simulink model "prach_shortFormat_fftShift"  (R2023b)
settings: Solver=FixedStepDiscrete  StartTime=0.0  StopTime=prach_short.SimulationTime  FixedStep=1  RelTol=1e-3  EnableMultiTasking=on
PreLoadFcn:
  | warning off Simulink:Commands:SetParamLinkChangeWarn
  | warning off Simulink:Commands:LoadMdlParameterizedLink
  | warning off Simulink:SL_SetParamLinkChangeWarn
  | warning off Simulink:SL_LoadMdlParameterizedLink
  | setup_prach_shortFormat;
InitFcn:
  | setup_prach_shortFormat;
StopFcn:
  | prach_post_run_script
values from neighbouring files (symbols this model uses):
  ConfigTable = [16 1 9,20,20,20,20,20,20,20,20,20 0 2 6 2 4 ... (first row only)    [ConfigIndexTable.m]
  NTxAnts = 4    [setup_prach_shortFormat.m]    (also in setup_prach_shortFormat_fftShift.m)
undefined symbols (not defined in the file or in its folder): AdvDSPBChannelOutDisplay, AdvDSPBDMemDisplay, BW, ControlDecode, display, dpoly, dspba, dspba_ChannelInVis, dspba_ChannelOutVis, dspba_internal_get_channel_ports, evalAionMaskParam, latency, PRACH_CC, PRACH_regs, prach_short, PrachLib, PrachLib_FFTshift, primtype, RemoveCP, Stream2BlockConv, UseDontCare, value, waveconfig
libraries: DSPBAPrim x397, DSPBAControl x16, DSPBAModelBus x7, DSPBABase x5, DSPBAUtilities x5, simulink x2, DSPBAVectorUtil x1, DspbAdvFftLibrary x1
(part 2 of 5)

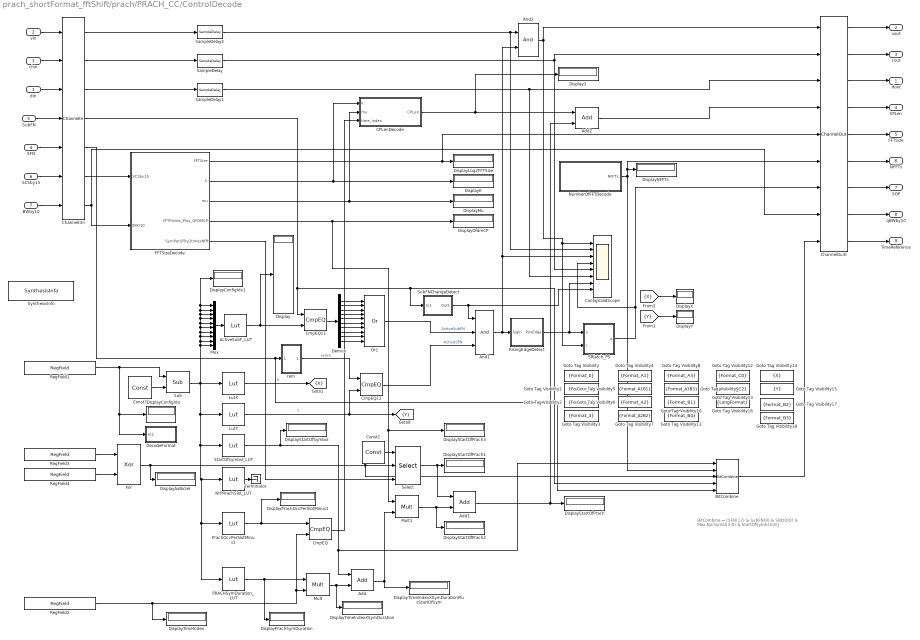
== system prach_shortFormat_fftShift/prach/PRACH_CC/ControlDecode ==
  note: BitCombine = [SFN(12) & SubFN(8) & SlotID(0) & Max.No.Symbl(3:0) & StartOfSymb(3:0)]
  din : Inport
  vin : Inport  Port=2
  chin : Inport  Port=3
  SFN : Inport  Port=4
  SubFN : Inport  Port=5
  SCSby15 : Inport  Port=6
  BWby10 : Inport  Port=7
  ActiveSubF_LUT : DSPBAPrim/Lut  primtype=lut  nInputs=1  nOutputs=1  omode=Inherit via internal rule  otype=sfix(16)  scale=2^-15  rndmethod=Unbiased  factor=1  satmethod=Symmetric  shift_vec=[0 1 2 -1]  value=ConfigTable(:,3:12)  inPortNames=[' '; ' ';]  outPortNames=[' ']  dspbaimage=dspba_prim.svg  text=fprintf('LUT');  style=Optimised  visibilities=8 + 1024  floatPrecision=float32_m23  version=20211007
  Add : DSPBAPrim/Add  primtype=add  nInputs=evalAionMaskParam(gcb,'value',1)  nOutputs=1  omode=Inherit via internal rule with word growth  otype=sfix(16)  scale=2^-15  rndmethod=Unbiased  factor=1  satmethod=Symmetric  shift_vec=[0 1 2 -1]  value=2  inPortNames=[' '; ' ';]  outPortNames=[' ']  dspbaimage=dspba_prim.svg  text=fprintf('+');  style=Optimised  visibilities=1032+2^17+2^18+2^19  genFPC=off  floatRounding=correct  advOptions=[]  version=20211007
  Add1 : DSPBAPrim/Add  primtype=add  nInputs=evalAionMaskParam(gcb,'value',1)  nOutputs=1  omode=Inherit via internal rule with word growth  otype=sfix(16)  scale=2^-15  rndmethod=Unbiased  factor=1  satmethod=Symmetric  shift_vec=[0 1 2 -1]  value=2  inPortNames=[' '; ' ';]  outPortNames=[' ']  dspbaimage=dspba_prim.svg  text=fprintf('+');  style=Optimised  visibilities=1032+2^17+2^18+2^19  genFPC=off  floatRounding=correct  advOptions=[]  version=20211007
  Add2 : DSPBAPrim/Add  primtype=add  nInputs=evalAionMaskParam(gcb,'value',1)  nOutputs=1  omode=Inherit via internal rule with word growth  otype=sfix(16)  scale=2^-15  rndmethod=Unbiased  factor=1  satmethod=Symmetric  shift_vec=[0 1 2 -1]  value=2  inPortNames=[' '; ' ';]  outPortNames=[' ']  dspbaimage=dspba_prim.svg  text=fprintf('+');  style=Optimised  visibilities=1032+2^17+2^18+2^19  genFPC=off  floatRounding=correct  advOptions=[]  version=20211007
  And1 : DSPBAPrim/And  primtype=and  nInputs=3  nOutputs=1  omode=Inherit via internal rule  otype=sfix(16)  scale=2^-15  rndmethod=Unbiased  factor=1  satmethod=Symmetric  shift_vec=[0 1 2 -1]  value=0  inPortNames=[' '; ' '; ' '; ' '; ' '; ' '; ' '; ' '; ' '; ' '; ' '; ' '; ' '; ' '; ' '; ' '; ]  outPortNames=[' ']  dspbaimage=dspba_prim.svg  text=fprintf('&');  style=Optimised  visibilities=8+2  version=20211007
  And2 : DSPBAPrim/And  primtype=and  nInputs=2  nOutputs=1  omode=Inherit via internal rule  otype=sfix(16)  scale=2^-15  rndmethod=Unbiased  factor=1  satmethod=Symmetric  shift_vec=[0 1 2 -1]  value=0  inPortNames=[' '; ' '; ' '; ' '; ' '; ' '; ' '; ' '; ' '; ' '; ' '; ' '; ' '; ' '; ' '; ' '; ]  outPortNames=[' ']  dspbaimage=dspba_prim.svg  text=fprintf('&');  style=Optimised  visibilities=8+2  version=20211007
  BitCombine : DSPBAPrim/BitCombine  primtype=bitcombine  nInputs=5  nOutputs=1  omode=Inherit via internal rule  otype=sfix(16)  scale=2^-15  rndmethod=Unbiased  factor=1  satmethod=Symmetric  shift_vec=[0 1 2 -1]  value=0  inPortNames=['l'; 'h';]  outPortNames=[' ']  dspbaimage=dspba_prim.svg  text=fprintf('[h,l]');  style=Optimised  visibilities=8+2  version=20211007
  CPLenDecode : Subsystem
      mask Display:
      | color('w');
      | image('dspba_prim.jpg');
      | port_label('output',1,'CPLen*nAnt');
      | port_label('input',1,'k');
      | port_label('input',2,'mu');
      | port_label('input',3,'time_index');
  ChannelI3n : DSPBAPrim/ChannelIn  primtype=channelin  nInputs=dspba_internal_get_channel_ports(gcb)  nOutputs=dspba_internal_get_channel_ports(gcb)  omode=Inherit via internal rule  otype=sfix(16)  scale=2^-15  rndmethod=Unbiased  factor=1  satmethod=Symmetric  shift_vec=[0 1 2 -1]  value=5  inPortNames=['v'; 'c'; '0'; '1'; '2'; '3'; '4'; '5'; '6'; '7'; '8'; '9'; 'A'; 'B'; 'D'; 'E'; 'F'; 'G'; 'H'; 'I'; 'J'; 'K'; 'L'; 'M'; 'N'; 'O'; 'P'; 'Q'; 'R'; 'S'; 'T'; 'U'; 'W'; 'X'; 'Y'; 'Z']  outPortNames=['v'; 'c'; '0'; '1'; '2'; '3'; '4'; '5'; '6'; '7'; '8'; '9'; 'A'; 'B'; 'D'; 'E'; 'F'; 'G'; 'H'; 'I'; 'J'; 'K'; 'L'; 'M'; 'N'; 'O'; 'P'; 'Q'; 'R'; 'S'; 'T'; 'U'; 'W'; 'X'; 'Y'; 'Z']  dspbaimage=dspba_prim_channel_tall.svg  text=fprintf('In');  style=Optimised  dataSignals=5  foldingEnabled=off  channels=1  sampleRate=200  packetBeginPresent=off  packetBeginEnabled=off  visibilities=dspba_ChannelInVis(gcb)  scheduleOrigin=on  version=20211214
  ChannelOu3t : DSPBAPrim/ChannelOut  primtype=channelout  nInputs=dspba_internal_get_channel_ports(gcb)  nOutputs=dspba_internal_get_channel_ports(gcb)  omode=Inherit via internal rule  otype=sfix(16)  scale=2^-15  rndmethod=Unbiased  factor=1  satmethod=Symmetric  shift_vec=[0 1 2 -1]  value=7  inPortNames=['v'; 'c'; '0'; '1'; '2'; '3'; '4'; '5'; '6'; '7'; '8'; '9'; 'A'; 'B'; 'D'; 'E'; 'F'; 'G'; 'H'; 'I'; 'J'; 'K'; 'L'; 'M'; 'N'; 'O'; 'P'; 'Q'; 'R'; 'S'; 'T'; 'U'; 'W'; 'X'; 'Y'; 'Z']  outPortNames=['v'; 'c'; '0'; '1'; '2'; '3'; '4'; '5'; '6'; '7'; '8'; '9'; 'A'; 'B'; 'D'; 'E'; 'F'; 'G'; 'H'; 'I'; 'J'; 'K'; 'L'; 'M'; 'N'; 'O'; 'P'; 'Q'; 'R'; 'S'; 'T'; 'U'; 'W'; 'X'; 'Y'; 'Z']  dspbaimage=dspba_prim_channel_tall.svg  text=fprintf('Out%s', AdvDSPBChannelOutDisplay(latency));  style=Optimised  dataSignals=7  foldingEnabled=off  channels=1  sampleRate=200  packetBeginPresent=off  packetBeginEnabled=off  visibilities=dspba_ChannelOutVis(gcb)  latency=17  version=20211214
  CmpEQ : DSPBAPrim/CmpEQ  primtype=cmpeq  nInputs=2  nOutputs=1  omode=boolean  otype=sfix(16)  scale=2^-15  rndmethod=Unbiased  factor=1  satmethod=Symmetric  shift_vec=[0 1 2 -1]  value=0  inPortNames=[' '; ' ';]  outPortNames=[' ']  dspbaimage=dspba_prim.svg  text=fprintf('==');  style=Optimised  visibilities=0  advOptions=[]  version=20211007
  CmpEQ11 : DSPBAPrim/CmpEQ  primtype=cmpeq  nInputs=2  nOutputs=1  omode=boolean  otype=sfix(16)  scale=2^-15  rndmethod=Unbiased  factor=1  satmethod=Symmetric  shift_vec=[0 1 2 -1]  value=0  inPortNames=[' '; ' ';]  outPortNames=[' ']  dspbaimage=dspba_prim.svg  text=fprintf('==');  style=Optimised  visibilities=0  advOptions=[]  version=20211007
  CmpEQ12 : DSPBAPrim/CmpEQ  primtype=cmpeq  nInputs=2  nOutputs=1  omode=boolean  otype=sfix(16)  scale=2^-15  rndmethod=Unbiased  factor=1  satmethod=Symmetric  shift_vec=[0 1 2 -1]  value=0  inPortNames=[' '; ' ';]  outPortNames=[' ']  dspbaimage=dspba_prim.svg  text=fprintf('==');  style=Optimised  visibilities=0  advOptions=[]  version=20211007
  ConfigValidScope : Scope  NumInputPorts=8
  Const1 : DSPBAPrim/Const  primtype=const  nInputs=0  nOutputs=1  omode=Inherit via internal rule  otype=sfix(16)  scale=2^-15  rndmethod=Unbiased  factor=1  satmethod=Symmetric  shift_vec=[0 1 2 -1]  value=0  inPortNames=['+'; '+';]  outPortNames=[' ']  dspbaimage=dspba_prim.svg  text=fprintf('%s', num2str(value));  style=Optimised  visibilities=8 + 1024  floatPrecision=float32_m23  warnSaturation=on  version=20211007  SampleTime=inf
  Const3 : DSPBAPrim/Const  primtype=const  nInputs=0  nOutputs=1  omode=Inherit via internal rule  otype=sfix(16)  scale=2^-15  rndmethod=Unbiased  factor=1  satmethod=Symmetric  shift_vec=[0 1 2 -1]  value=67  inPortNames=['+'; '+';]  outPortNames=[' ']  dspbaimage=dspba_prim.svg  text=fprintf('%s', num2str(value));  style=Optimised  visibilities=8 + 1024  floatPrecision=float32_m23  warnSaturation=on  version=20211007  SampleTime=inf
  DecodeFormat : Subsystem
  Demux : Demux  Outputs=10
  Display : Display
  Display3 : Display
  DisplayAxBxSel : Display
  DisplayConfigIdx : Display
  DisplayConfigIdx1 : Display
  DisplayK : Display
  DisplayLog2FFTSize : Display
  DisplayMu : Display
  DisplayNFFTs : Display
  DisplayOfdmCP : Display
  DisplayPrachOccPerSlotMinus1 : Display
  DisplayPrachSymDuration : Display
  DisplayStartOfPrach{,1..3} (4 alike) : Display
  DisplayStartOfSymbol : Display
  DisplayTimeIndex : Display
  DisplayTimeIndexXSymDuration : Display
  DisplayTimeIndexXSymDurationPlusStartOfSym : Display
  DisplayX : Display
  DisplayY : Display
  FFTSizeDecode : Subsystem
      mask Display:
      | color('w');
      | image('dspba_prim.jpg');
      | port_label('output',1,'log2(FFT size)');
      | port_label('output',2,'k');
      | port_label('output',3,'mu');
      | port_label('output',4,'FFTPoints+OFDM_CP');
      | port_label('output',5,'SymPerSF/2*Nfft');
      | port_label('input',1,'SCS/15');
      | port_label('input',2,'BW/10');
  Goto Tag Visibility : GotoTagVisibility  GotoTag=Format_0
  Goto Tag Visibility1 : GotoTagVisibility  GotoTag=Format_1
  Goto Tag Visibility10 : GotoTagVisibility  GotoTag=Format_B1
  Goto Tag Visibility11 : GotoTagVisibility  GotoTag=Format_B4
  Goto Tag Visibility12 : GotoTagVisibility  GotoTag=Format_C0
  Goto Tag Visibility13 : GotoTagVisibility  GotoTag=Format_C2
  Goto Tag Visibility14 : GotoTagVisibility  GotoTag=X
  Goto Tag Visibility15 : GotoTagVisibility  GotoTag=Y
  Goto Tag Visibility16 : GotoTagVisibility  GotoTag=LongFormat
  Goto Tag Visibility17 : GotoTagVisibility  GotoTag=Format_B2
  Goto Tag Visibility18 : GotoTagVisibility  GotoTag=Format_B3
  Goto Tag Visibility2 : GotoTagVisibility  GotoTag=Format_2
  Goto Tag Visibility3 : GotoTagVisibility  GotoTag=Format_3
  Goto Tag Visibility4 : GotoTagVisibility  GotoTag=Format_A1
  Goto Tag Visibility5 : GotoTagVisibility  GotoTag=Format_A1B1
  Goto Tag Visibility6 : GotoTagVisibility  GotoTag=Format_A2
  Goto Tag Visibility7 : GotoTagVisibility  GotoTag=Format_A2B2
  Goto Tag Visibility8 : GotoTagVisibility  GotoTag=Format_A3
  Goto Tag Visibility9 : GotoTagVisibility  GotoTag=Format_A3B3
  LutX : DSPBAPrim/Lut  primtype=lut  nInputs=1  nOutputs=1  omode=Inherit via internal rule  otype=sfix(16)  scale=2^-15  rndmethod=Unbiased  factor=1  satmethod=Symmetric  shift_vec=[0 1 2 -1]  value=ConfigTable(:,1)  inPortNames=[' '; ' ';]  outPortNames=[' ']  dspbaimage=dspba_prim.svg  text=fprintf('LUT');  style=Optimised  visibilities=8 + 1024  floatPrecision=float32_m23  version=20211007
  LutY : DSPBAPrim/Lut  primtype=lut  nInputs=1  nOutputs=1  omode=Inherit via internal rule  otype=sfix(16)  scale=2^-15  rndmethod=Unbiased  factor=1  satmethod=Symmetric  shift_vec=[0 1 2 -1]  value=ConfigTable(:,2)  inPortNames=[' '; ' ';]  outPortNames=[' ']  dspbaimage=dspba_prim.svg  text=fprintf('LUT');  style=Optimised  visibilities=8 + 1024  floatPrecision=float32_m23  version=20211007
  Mult : DSPBAPrim/Mult  primtype=mult  nInputs=2  nOutputs=1  omode=Inherit via internal rule  otype=sfix(16)  scale=2^-15  rndmethod=Unbiased  factor=1  satmethod=Symmetric  shift_vec=[0 1 2 -1]  value=0  inPortNames=[' '; ' ';]  outPortNames=[' ']  dspbaimage=dspba_prim.svg  text=fprintf('X');  style=Optimised  visibilities=8+2^18+2^19  floatPrecision=float32_m23  floatRounding=correct  advOptions=[]  version=20211007
  Mult1 : DSPBAPrim/Mult  primtype=mult  nInputs=2  nOutputs=1  omode=Inherit via internal rule  otype=sfix(16)  scale=2^-15  rndmethod=Unbiased  factor=1  satmethod=Symmetric  shift_vec=[0 1 2 -1]  value=0  inPortNames=[' '; ' ';]  outPortNames=[' ']  dspbaimage=dspba_prim.svg  text=fprintf('X');  style=Optimised  visibilities=8+2^18+2^19  floatPrecision=float32_m23  floatRounding=correct  advOptions=[]  version=20211007
  Mux : Mux  Inputs=10
  NrPRrachSlot_LUT : DSPBAPrim/Lut  primtype=lut  nInputs=1  nOutputs=1  omode=Inherit via internal rule  otype=sfix(16)  scale=2^-15  rndmethod=Unbiased  factor=1  satmethod=Symmetric  shift_vec=[0 1 2 -1]  value=ConfigTable(:,14)  inPortNames=[' '; ' ';]  outPortNames=[' ']  dspbaimage=dspba_prim.svg  text=fprintf('LUT');  style=Optimised  visibilities=8 + 1024  floatPrecision=float32_m23  version=20211007
  NumberOfFFTDecode : Subsystem
      mask Display:
      | color('w');
      | image('dspba_prim.jpg');
      | port_label('output',1,'Number of FFTs');
  Or1 : DSPBAPrim/Or  primtype=or  nInputs=10  nOutputs=1  omode=Inherit via internal rule  otype=sfix(16)  scale=2^-15  rndmethod=Unbiased  factor=1  satmethod=Symmetric  shift_vec=[0 1 2 -1]  value=0  inPortNames=[' '; ' '; ' '; ' '; ' '; ' '; ' '; ' '; ' '; ' '; ' '; ' '; ' '; ' '; ' '; ' '; ]  outPortNames=[' ']  dspbaimage=dspba_prim.svg  text=fprintf('|');  style=Optimised  visibilities=8+2  version=20211007
  PRACHSymDuration_LUT : DSPBAPrim/Lut  primtype=lut  nInputs=1  nOutputs=1  omode=Inherit via internal rule  otype=sfix(16)  scale=2^-15  rndmethod=Unbiased  factor=1  satmethod=Symmetric  shift_vec=[0 1 2 -1]  value=ConfigTable(:,16)  inPortNames=[' '; ' ';]  outPortNames=[' ']  dspbaimage=dspba_prim.svg  text=fprintf('LUT');  style=Optimised  visibilities=8 + 1024  floatPrecision=float32_m23  version=20211007
  PrachOccPerSlotMinus1 : DSPBAPrim/Lut  primtype=lut  nInputs=1  nOutputs=1  omode=Inherit via internal rule  otype=sfix(16)  scale=2^-15  rndmethod=Unbiased  factor=1  satmethod=Symmetric  shift_vec=[0 1 2 -1]  value=ConfigTable(:,15)-1  inPortNames=[' '; ' ';]  outPortNames=[' ']  dspbaimage=dspba_prim.svg  text=fprintf('LUT');  style=Optimised  visibilities=8 + 1024  floatPrecision=float32_m23  version=20211007
  RegField1 : DSPBAModelBus/RegField  reg_name=PRACH_regs(InstanceNumber).PRACH_config_index_addr  reg_rwmode=Read/Write  reg_msb=7  reg_lsb=0  reg_mode=Specify via dialog  reg_type=uint(8)  reg_scale=2^0  reg_init=PRACH_regs(InstanceNumber).PRACH_config_index  reg_desc=PRACH_regs(InstanceNumber).PRACH_config_index_string  reg_modal=off  reg_desc0=0  reg_desc1=0  reg_desc2=0  reg_desc3=0  reg_desc4=0  reg_desc5=0  reg_desc6=0  reg_desc7=0  reg_addr=8  SampleTime=-1  version=20090407
  RegField2 : DSPBAModelBus/RegField  reg_name=PRACH_regs(InstanceNumber).PRACH_time_index_addr  reg_rwmode=Read/Write  reg_msb=2  reg_lsb=0  reg_mode=Specify via dialog  reg_type=uint(3)  reg_scale=2^0  reg_init=PRACH_regs(InstanceNumber).PRACH_time_index  reg_desc=PRACH_regs(InstanceNumber).PRACH_time_index_string  reg_modal=off  reg_desc0=0  reg_desc1=0  reg_desc2=0  reg_desc3=0  reg_desc4=0  reg_desc5=0  reg_desc6=0  reg_desc7=0  reg_addr=9  SampleTime=-1  version=20090407
  RegField3 : DSPBAModelBus/RegField  reg_name=PRACH_regs(InstanceNumber).PRACH_NRPRACHSlot_addr  reg_rwmode=Read/Write  reg_msb=0  reg_lsb=0  reg_mode=Specify via dialog  reg_type=uint(1)  reg_scale=2^0  reg_init=PRACH_regs(InstanceNumber).PRACH_NRPRACHSlot  reg_desc=PRACH_regs(InstanceNumber).PRACH_NRPRACHSlot_string  reg_modal=off  reg_desc0=0  reg_desc1=0  reg_desc2=0  reg_desc3=0  reg_desc4=0  reg_desc5=0  reg_desc6=0  reg_desc7=0  reg_addr=10  SampleTime=-1  version=20090407
  RegField4 : DSPBAModelBus/RegField  reg_name=PRACH_regs(InstanceNumber).PRACH_ActivePRACHSlot_addr  reg_rwmode=Read/Write  reg_msb=0  reg_lsb=0  reg_mode=Specify via dialog  reg_type=uint(1)  reg_scale=2^0  reg_init=PRACH_regs(InstanceNumber).PRACH_ActivePRACHSlot  reg_desc=PRACH_regs(InstanceNumber).PRACH_ActivePRACHSlot_string  reg_modal=off  reg_desc0=0  reg_desc1=0  reg_desc2=0  reg_desc3=0  reg_desc4=0  reg_desc5=0  reg_desc6=0  reg_desc7=0  reg_addr=11  SampleTime=-1  version=20090407
  RisingEdgeDetect : Subsystem
  SRlatch_PS : Subsystem  AncestorBlock=DSPBAControl/SRlatch_PS  mask(SetResetLatchPrioritySet){}
      mask help: DSP Builder offers two single-cycle latency latch subsystems for common operations for the valid signal, latching with set and reset. The SRlatch block gives priority to the reset input signal; the SRlatch_PS block gives priority to the set input signal. In both blocks, if set and reset inputs are both zero the current output state is maintained.
      mask Help: helpview(dspba.GetHelp('SRlatch_PS'));
      mask Display:
      | color('w');
      | image('dspba_prim_masked.png');
      | fprintf('SRlatch\nPriority\nSet');
      | port_label('input',1,'s');
      | port_label('input',2,'r');
      | port_label('output',1,'q');
  SampleDelay : DSPBAPrim/SampleDelay  primtype=sampdelay  nInputs=1  nOutputs=1  omode=Inherit via internal rule  otype=sfix(16)  scale=2^-15  rndmethod=Unbiased  factor=1  satmethod=Symmetric  shift_vec=[0 1 2 -1]  floatPrecision=float32_m23  value=1  inPortNames=[' '; ' ';]  outPortNames=[' ']  dspbaimage=dspba_prim.svg  text=dpoly(1, eye(1,value+1), 'z')  style=Optimised  visibilities=8 + 1024 + 2^17 + 2^18  flexible=off  slackgroup=0  augmented=0  version=20211007  advOptions=[]
  SampleDelay1 : DSPBAPrim/SampleDelay  primtype=sampdelay  nInputs=1  nOutputs=1  omode=Inherit via internal rule  otype=sfix(16)  scale=2^-15  rndmethod=Unbiased  factor=1  satmethod=Symmetric  shift_vec=[0 1 2 -1]  floatPrecision=float32_m23  value=1  inPortNames=[' '; ' ';]  outPortNames=[' ']  dspbaimage=dspba_prim.svg  text=dpoly(1, eye(1,value+1), 'z')  style=Optimised  visibilities=8 + 1024 + 2^17 + 2^18  flexible=off  slackgroup=0  augmented=0  version=20211007  advOptions=[]
  SampleDelay2 : DSPBAPrim/SampleDelay  primtype=sampdelay  nInputs=1  nOutputs=1  omode=Inherit via internal rule  otype=sfix(16)  scale=2^-15  rndmethod=Unbiased  factor=1  satmethod=Symmetric  shift_vec=[0 1 2 -1]  floatPrecision=float32_m23  value=1  inPortNames=[' '; ' ';]  outPortNames=[' ']  dspbaimage=dspba_prim.svg  text=dpoly(1, eye(1,value+1), 'z')  style=Optimised  visibilities=8 + 1024 + 2^17 + 2^18  flexible=off  slackgroup=0  augmented=0  version=20211007  advOptions=[]
  Select : DSPBAPrim/Select  primtype=select  nInputs=str2num(get_param(gcb,'value'))*2+1  nOutputs=1  omode=Inherit via internal rule  otype=sfix(16)  scale=2^-15  rndmethod=Unbiased  factor=1  satmethod=Symmetric  shift_vec=[0 1 2 -1]  value=1  inPortNames=['d'; '0'; 'a'; '1'; 'b'; '2'; 'c'; '3'; 'd'; '4'; 'e'; '5'; 'f'; '6'; 'g'; '7'; 'h'; '8'; 'i'; '9'; 'j']  outPortNames=[' ']  dspbaimage=dspba_prim_tall.svg  text=fprintf('%s', primtype);  style=Optimised  visibilities=8 + 1024  version=20211007
  StartOfSymbol_LUT : DSPBAPrim/Lut  primtype=lut  nInputs=1  nOutputs=1  omode=Inherit via internal rule  otype=sfix(16)  scale=2^-15  rndmethod=Unbiased  factor=1  satmethod=Symmetric  shift_vec=[0 1 2 -1]  value=ConfigTable(:,13)  inPortNames=[' '; ' ';]  outPortNames=[' ']  dspbaimage=dspba_prim.svg  text=fprintf('LUT');  style=Optimised  visibilities=8 + 1024  floatPrecision=float32_m23  version=20211007
  Sub : DSPBAPrim/Sub  primtype=sub  nInputs=2  nOutputs=1  omode=Specify via dialog  otype=uint(8)  scale=1  rndmethod=Unbiased  factor=1  satmethod=Symmetric  shift_vec=[0 1 2 -1]  value=0  inPortNames=['+'; '-';]  outPortNames=[' ']  dspbaimage=dspba_prim.svg  text=fprintf('-');  style=Optimised  visibilities=8+2^17+2^18  floatRounding=correct  advOptions=[]  version=20211007
  SubFNChangeDetect : Subsystem
  SynthesisInfo : DSPBAPrim/SynthesisInfo  primtype=synthinfo  nInputs=0  nOutputs=0  omode=Inherit via internal rule  otype=sfix(16)  scale=2^-15  rndmethod=Truncate  factor=1  satmethod=Symmetric  shift_vec=[0 1 2 -1]  value=99  inPortNames=[' '; ' ';]  outPortNames=[' ']  dspbaimage=dspba_prim_ctrl.jpg  text=fprintf('Style=%s', style);  style=Scheduled  visibilities=2^17+2^18+2^19+2^20+2^21+2^22+2^23+2^24  constraintPair=None  constraintRelation=>  constraintLimit=2  modelRefSign=+  modelRef=''  showSchedule=off  simulationMode=Use Global Value  resetMinimization=Conditional - On for ChannelIn/Out only  version=20220106
  Terminator : Terminator
  Xor : DSPBAPrim/Xor  primtype=xor  nInputs=2  nOutputs=1  omode=Inherit via internal rule  otype=sfix(16)  scale=2^-15  rndmethod=Unbiased  factor=1  satmethod=Symmetric  shift_vec=[0 1 2 -1]  value=0  inPortNames=[' '; ' '; ' '; ' '; ' '; ' '; ' '; ' '; ' '; ' '; ' '; ' '; ' '; ' '; ' '; ' '; ]  outPortNames=[' ']  dspbaimage=dspba_prim.svg  text=fprintf('^');  style=Optimised  visibilities=8+2  version=20211007
  rem : Subsystem
  dout : Outport  VectorParamsAs1DForOutWhenUnconnected=off
  vout : Outport  Port=2  VectorParamsAs1DForOutWhenUnconnected=off
  cout : Outport  Port=3  VectorParamsAs1DForOutWhenUnconnected=off
  CPLen : Outport  Port=4  VectorParamsAs1DForOutWhenUnconnected=off
  FFTSize : Outport  Port=5  VectorParamsAs1DForOutWhenUnconnected=off
  NFFTs : Outport  Port=6  VectorParamsAs1DForOutWhenUnconnected=off
  SOP : Outport  Port=7  VectorParamsAs1DForOutWhenUnconnected=off
  qBWby10 : Outport  Port=8  VectorParamsAs1DForOutWhenUnconnected=off
  TimeReference : Outport  Port=9  VectorParamsAs1DForOutWhenUnconnected=off
  tag scope: X=scoped, Y=scoped
  wires:
  LutY/1 -> [Y], CmpEQ12/2  "Y"
  LutX/1 -> [X]  "X"
  Mux/1 -> ActiveSubF_LUT/1
  ActiveSubF_LUT/1 -> CmpEQ11/2, Display/1
  ChannelI3n/3 -> SampleDelay1/1
  ChannelI3n/4 -> SubFNChangeDetect/1(In1), BitCombine/4, CmpEQ11/1
  din/1 -> ChannelI3n/3
  chin/1 -> ChannelI3n/2
  vin/1 -> ChannelI3n/1
  ChannelI3n/2 -> SampleDelay/1
  ChannelOu3t/3 -> dout/1
  ChannelOu3t/2 -> cout/1
  ChannelOu3t/1 -> vout/1
  SampleDelay2/1 -> ConfigValidScope/2, And2/1
  RegField1/1 -> DisplayConfigIdx/1, DecodeFormat/1(In1), Sub/1
  ChannelI3n/5 -> BitCombine/5, rem/1(SFN)
  rem/1(rem) -> CmpEQ12/1  "remX"
  CmpEQ12/1 -> And1/3  "ActiveSFN"
  And2/1 -> SRlatch_PS/2(r), ConfigValidScope/1, ChannelOu3t/1
  Demux/1 -> Or1/1
  Demux/2 -> Or1/2
  Demux/3 -> Or1/3
  Demux/4 -> Or1/4
  Demux/5 -> Or1/5
  Demux/6 -> Or1/6
  Demux/7 -> Or1/7
  Demux/8 -> Or1/8
  Demux/9 -> Or1/9
  Demux/10 -> Or1/10
  CmpEQ11/1 -> Demux/1
  Sub/1 -> LutX/1, PRACHSymDuration_LUT/1, PrachOccPerSlotMinus1/1, NrPRrachSlot_LUT/1, StartOfSymbol_LUT/1, LutY/1, DisplayConfigIdx1/1, Mux/1, Mux/2, Mux/3, Mux/4, Mux/5, Mux/6, Mux/7, Mux/8, Mux/9, Mux/10
  Const3/1 -> Sub/2
  SubFN/1 -> ChannelI3n/4
  SFN/1 -> ChannelI3n/5
  CPLenDecode/1(CPLen) -> Add2/1, Display3/1
  ChannelOu3t/4 -> CPLen/1
  ChannelOu3t/5 -> FFTSize/1
  SCSby15/1 -> ChannelI3n/6
  BWby10/1 -> ChannelI3n/7
  ChannelI3n/6 -> FFTSizeDecode/1(SCSby15)
  ChannelI3n/7 -> FFTSizeDecode/2(BW/10), ChannelOu3t/8
  FFTSizeDecode/2(k) -> CPLenDecode/1(k), DisplayK/1
  FFTSizeDecode/3(mu) -> CPLenDecode/2(mu), DisplayMu/1
  [X] -> DisplayX/1
  [Y] -> DisplayY/1
  NumberOfFFTDecode/1(NFFTs) -> ChannelOu3t/6, DisplayNFFTs/1, BitCombine/2
  ChannelOu3t/6 -> NFFTs/1
  And1/1 -> RisingEdgeDetect/1(SigIn), And2/2, ConfigValidScope/3
  Or1/1 -> And1/2  "ActiveSubFN"
  ChannelOu3t/7 -> SOP/1
  RisingEdgeDetect/1(PosEdge) -> ConfigValidScope/7, SRlatch_PS/1(s)
  FFTSizeDecode/1(FFTSize) -> DisplayLog2FFTSize/1, ChannelOu3t/5
  FFTSizeDecode/4(FFTPoints_Plus_OFDMCP) -> Mult1/1, DisplayStartOfPrach3/1, DisplayOfdmCP/1
  RegField2/1 -> DisplayTimeIndex/1, CmpEQ/2, Mult/2
  PRACHSymDuration_LUT/1 -> DisplayPrachSymDuration/1, Mult/1
  Mult/1 -> DisplayTimeIndexXSymDuration/1, Add/2
  StartOfSymbol_LUT/1 -> DisplayStartOfSymbol/1, BitCombine/1, Add/1
  Add/1 -> Mult1/2, DisplayTimeIndexXSymDurationPlusStartOfSym/1
  Mult1/1 -> DisplayStartOfPrach2/1, Add1/2
  FFTSizeDecode/5(SymPerSFby2timesNfft) -> Select/3
  RegField3/1 -> Xor/1
  RegField4/1 -> Xor/2
  Select/1 -> DisplayStartOfPrach1/1, Add1/1
  Xor/1 -> DisplayAxBxSel/1, BitCombine/3, Select/2
  Const1/1 -> Select/1
  Add1/1 -> Add2/2, DisplayStartOfPrach/1
  Add2/1 -> ChannelOu3t/4
  ChannelOu3t/8 -> qBWby10/1
  SRlatch_PS/1(q) -> ChannelOu3t/7, ConfigValidScope/4
  CmpEQ/1 -> CPLenDecode/3(time_index)
  NrPRrachSlot_LUT/1 -> Terminator/1
  PrachOccPerSlotMinus1/1 -> CmpEQ/1, DisplayPrachOccPerSlotMinus1/1
  BitCombine/1 -> ChannelOu3t/9
  ChannelOu3t/9 -> TimeReference/1
  SubFNChangeDetect/1(Out1) -> ConfigValidScope/8, And1/1
  SampleDelay/1 -> ChannelOu3t/2, ConfigValidScope/5
  SampleDelay1/1 -> ConfigValidScope/6, ChannelOu3t/3
  ChannelI3n/1 -> SampleDelay2/1

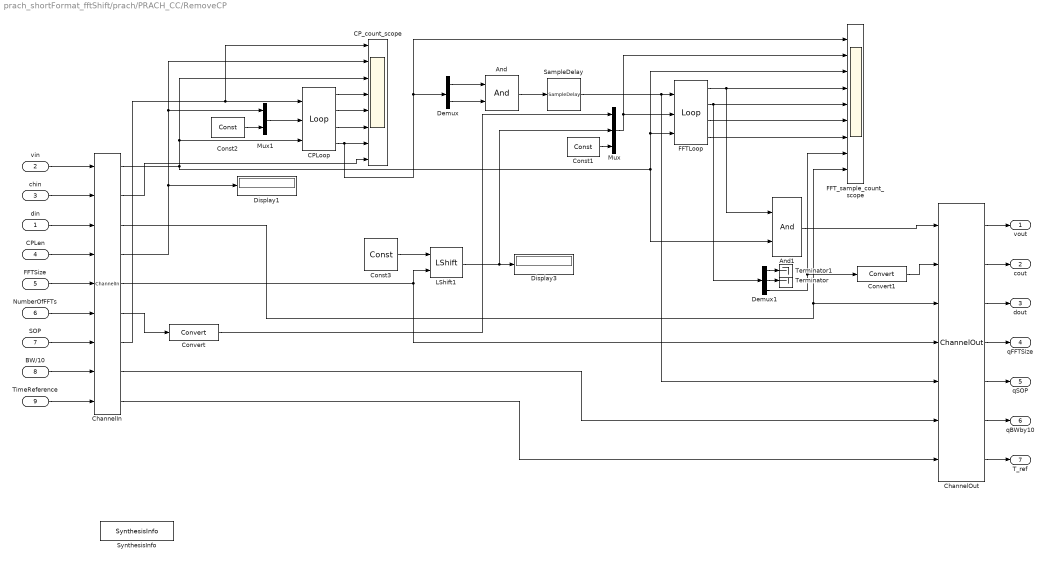
== system prach_shortFormat_fftShift/prach/PRACH_CC/RemoveCP ==
  din : Inport
  vin : Inport  Port=2
  chin : Inport  Port=3
  CPLen : Inport  Port=4
  FFTSize : Inport  Port=5
  NumberOfFFTs : Inport  Port=6
  SOP : Inport  Port=7
  BW/10 : Inport  Port=8
  TimeReference : Inport  Port=9
  And : DSPBAPrim/And  primtype=and  nInputs=2  nOutputs=1  omode=Inherit via internal rule  otype=sfix(16)  scale=2^-15  rndmethod=Unbiased  factor=1  satmethod=Symmetric  shift_vec=[0 1 2 -1]  value=0  inPortNames=[' '; ' '; ' '; ' '; ' '; ' '; ' '; ' '; ' '; ' '; ' '; ' '; ' '; ' '; ' '; ' '; ]  outPortNames=[' ']  dspbaimage=dspba_prim.svg  text=fprintf('&');  style=Optimised  visibilities=8+2  version=20211007
  And1 : DSPBAPrim/And  primtype=and  nInputs=2  nOutputs=1  omode=Inherit via internal rule  otype=sfix(16)  scale=2^-15  rndmethod=Unbiased  factor=1  satmethod=Symmetric  shift_vec=[0 1 2 -1]  value=0  inPortNames=[' '; ' '; ' '; ' '; ' '; ' '; ' '; ' '; ' '; ' '; ' '; ' '; ' '; ' '; ' '; ' '; ]  outPortNames=[' ']  dspbaimage=dspba_prim.svg  text=fprintf('&');  style=Optimised  visibilities=8+2  version=20211007
  CPLoop : DSPBAPrim/Loop  primtype=loop  nInputs=3  nOutputs=4  omode=Inherit via internal rule  otype=sfix(16)  scale=2^-15  rndmethod=Unbiased  factor=1  satmethod=Symmetric  shift_vec=[0 1 2 -1]  value=[zeros(16, 1)]  inPortNames=['g'; 'c'; 'e']  outPortNames=['v'; 'q'; 'f'; 'l']  dspbaimage=dspba_prim_tall.svg  text=fprintf('loop');  style=Optimised  visibilities=0  version=20211007
  CP_count_scope : Scope  NumInputPorts=8
  ChannelIn : DSPBAPrim/ChannelIn  primtype=channelin  nInputs=dspba_internal_get_channel_ports(gcb)  nOutputs=dspba_internal_get_channel_ports(gcb)  omode=Inherit via internal rule  otype=sfix(16)  scale=2^-15  rndmethod=Unbiased  factor=1  satmethod=Symmetric  shift_vec=[0 1 2 -1]  value=7  inPortNames=['v'; 'c'; '0'; '1'; '2'; '3'; '4'; '5'; '6'; '7'; '8'; '9'; 'A'; 'B'; 'D'; 'E'; 'F'; 'G'; 'H'; 'I'; 'J'; 'K'; 'L'; 'M'; 'N'; 'O'; 'P'; 'Q'; 'R'; 'S'; 'T'; 'U'; 'W'; 'X'; 'Y'; 'Z']  outPortNames=['v'; 'c'; '0'; '1'; '2'; '3'; '4'; '5'; '6'; '7'; '8'; '9'; 'A'; 'B'; 'D'; 'E'; 'F'; 'G'; 'H'; 'I'; 'J'; 'K'; 'L'; 'M'; 'N'; 'O'; 'P'; 'Q'; 'R'; 'S'; 'T'; 'U'; 'W'; 'X'; 'Y'; 'Z']  dspbaimage=dspba_prim_channel_tall.svg  text=fprintf('In');  style=Optimised  dataSignals=7  foldingEnabled=off  channels=1  sampleRate=200  packetBeginPresent=off  packetBeginEnabled=off  visibilities=dspba_ChannelInVis(gcb)  scheduleOrigin=on  version=20211214
  ChannelOut : DSPBAPrim/ChannelOut  primtype=channelout  nInputs=dspba_internal_get_channel_ports(gcb)  nOutputs=dspba_internal_get_channel_ports(gcb)  omode=Inherit via internal rule  otype=sfix(16)  scale=2^-15  rndmethod=Unbiased  factor=1  satmethod=Symmetric  shift_vec=[0 1 2 -1]  value=5  inPortNames=['v'; 'c'; '0'; '1'; '2'; '3'; '4'; '5'; '6'; '7'; '8'; '9'; 'A'; 'B'; 'D'; 'E'; 'F'; 'G'; 'H'; 'I'; 'J'; 'K'; 'L'; 'M'; 'N'; 'O'; 'P'; 'Q'; 'R'; 'S'; 'T'; 'U'; 'W'; 'X'; 'Y'; 'Z']  outPortNames=['v'; 'c'; '0'; '1'; '2'; '3'; '4'; '5'; '6'; '7'; '8'; '9'; 'A'; 'B'; 'D'; 'E'; 'F'; 'G'; 'H'; 'I'; 'J'; 'K'; 'L'; 'M'; 'N'; 'O'; 'P'; 'Q'; 'R'; 'S'; 'T'; 'U'; 'W'; 'X'; 'Y'; 'Z']  dspbaimage=dspba_prim_channel_tall.svg  text=fprintf('Out%s', AdvDSPBChannelOutDisplay(latency));  style=Optimised  dataSignals=5  foldingEnabled=off  channels=1  sampleRate=200  packetBeginPresent=off  packetBeginEnabled=off  visibilities=dspba_ChannelOutVis(gcb)  latency=2  version=20211214
  Const1 : DSPBAPrim/Const  primtype=const  nInputs=0  nOutputs=1  omode=Inherit via back propagation  otype=sfix(16)  scale=2^-15  rndmethod=Unbiased  factor=1  satmethod=Symmetric  shift_vec=[0 1 2 -1]  value=NAnts  inPortNames=['+'; '+';]  outPortNames=[' ']  dspbaimage=dspba_prim.svg  text=fprintf('%s', num2str(value));  style=Optimised  visibilities=8 + 1024  floatPrecision=float32_m23  warnSaturation=on  version=20211007  SampleTime=inf
  Const2 : DSPBAPrim/Const  primtype=const  nInputs=0  nOutputs=1  omode=Inherit via back propagation  otype=sfix(16)  scale=2^-15  rndmethod=Unbiased  factor=1  satmethod=Symmetric  shift_vec=[0 1 2 -1]  value=NAnts  inPortNames=['+'; '+';]  outPortNames=[' ']  dspbaimage=dspba_prim.svg  text=fprintf('%s', num2str(value));  style=Optimised  visibilities=8 + 1024  floatPrecision=float32_m23  warnSaturation=on  version=20211007  SampleTime=inf
  Const3 : DSPBAPrim/Const  primtype=const  nInputs=0  nOutputs=1  omode=Inherit via internal rule  otype=sfix(16)  scale=2^-15  rndmethod=Unbiased  factor=1  satmethod=Symmetric  shift_vec=[0 1 2 -1]  value=1  inPortNames=['+'; '+';]  outPortNames=[' ']  dspbaimage=dspba_prim.svg  text=fprintf('%s', num2str(value));  style=Optimised  visibilities=8 + 1024  floatPrecision=float32_m23  warnSaturation=on  version=20211007  SampleTime=inf
  Convert : DSPBAPrim/Convert  primtype=convert  nInputs=1  nOutputs=1  omode=Inherit via back propagation  otype=sfix(16)  scale=2^-15  rndmethod=Truncate  factor=1  satmethod=None  shift_vec=[0 1 2 -1]  value=round([0:255]/17)  inPortNames=[' '; ' ';]  outPortNames=[' '; 'c']  dspbaimage=dspba_prim_wide.svg  text=fprintf('convert');  style=Optimised  visibilities=8+64+256+2^17  clipdetect=off  floatPrecision=float32_m23  advOptions=[]  version=20211007
  Convert1 : DSPBAPrim/Convert  primtype=convert  nInputs=1  nOutputs=1  omode=Specify via dialog  otype=ufix(8)  scale=1  rndmethod=Truncate  factor=1  satmethod=None  shift_vec=[0 1 2 -1]  value=round([0:255]/17)  inPortNames=[' '; ' ';]  outPortNames=[' '; 'c']  dspbaimage=dspba_prim_wide.svg  text=fprintf('convert');  style=Optimised  visibilities=8+64+256+2^17  clipdetect=off  floatPrecision=float32_m23  advOptions=[]  version=20211007
  Demux : Demux  Outputs=2
  Demux1 : Demux  Outputs=3
  Display1 : Display
  Display3 : Display
  FFTLoop : DSPBAPrim/Loop  primtype=loop  nInputs=3  nOutputs=4  omode=Inherit via internal rule  otype=sfix(16)  scale=2^-15  rndmethod=Unbiased  factor=1  satmethod=Symmetric  shift_vec=[0 1 2 -1]  value=[zeros(16, 1)]  inPortNames=['g'; 'c'; 'e']  outPortNames=['v'; 'q'; 'f'; 'l']  dspbaimage=dspba_prim_tall.svg  text=fprintf('loop');  style=Optimised  visibilities=0  version=20211007
  FFT_sample_count_scope : Scope  NumInputPorts=9
  LShift1 : DSPBAPrim/LShift  primtype=lshift  nInputs=2  nOutputs=1  omode=Specify via dialog  otype=ufix(log2(prach_short.Nfft)+1)  scale=1  rndmethod=Unbiased  factor=1  satmethod=Symmetric  shift_vec=[0 1 2 -1]  value=0  inPortNames=['a'; 'b';]  outPortNames=[' ']  dspbaimage=dspba_prim.svg  text=fprintf('a << b');  style=Optimised  visibilities=8  version=20211007
  Mux : Mux  Inputs=3
  Mux1 : Mux  Inputs=2
  SampleDelay : DSPBAPrim/SampleDelay  primtype=sampdelay  nInputs=1  nOutputs=1  omode=Inherit via internal rule  otype=sfix(16)  scale=2^-15  rndmethod=Unbiased  factor=1  satmethod=Symmetric  shift_vec=[0 1 2 -1]  floatPrecision=float32_m23  value=1  inPortNames=[' '; ' ';]  outPortNames=[' ']  dspbaimage=dspba_prim.svg  text=dpoly(1, eye(1,value+1), 'z')  style=Optimised  visibilities=8 + 1024 + 2^17 + 2^18  flexible=off  slackgroup=0  augmented=0  version=20211007  advOptions=[]
  SynthesisInfo : DSPBAPrim/SynthesisInfo  primtype=synthinfo  nInputs=0  nOutputs=0  omode=Inherit via internal rule  otype=sfix(16)  scale=2^-15  rndmethod=Truncate  factor=1  satmethod=Symmetric  shift_vec=[0 1 2 -1]  value=99  inPortNames=[' '; ' ';]  outPortNames=[' ']  dspbaimage=dspba_prim_ctrl.jpg  text=fprintf('Style=%s', style);  style=Scheduled  visibilities=2^17+2^18+2^19+2^20+2^21+2^22+2^23+2^24  constraintPair=None  constraintRelation=>  constraintLimit=6  modelRefSign=+  modelRef=''  showSchedule=off  simulationMode=Use Global Value  resetMinimization=Conditional - On for ChannelIn/Out only  version=20220106
  Terminator : Terminator
  Terminator1 : Terminator
  vout : Outport  VectorParamsAs1DForOutWhenUnconnected=off
  cout : Outport  Port=2  VectorParamsAs1DForOutWhenUnconnected=off
  dout : Outport  Port=3  VectorParamsAs1DForOutWhenUnconnected=off
  qFFTSize : Outport  Port=4  VectorParamsAs1DForOutWhenUnconnected=off
  qSOP : Outport  Port=5  VectorParamsAs1DForOutWhenUnconnected=off
  qBWby10 : Outport  Port=6  VectorParamsAs1DForOutWhenUnconnected=off
  T_ref : Outport  Port=7  VectorParamsAs1DForOutWhenUnconnected=off
  wires:
  ChannelIn/1 -> FFT_sample_count_scope/3, FFTLoop/3, And1/2, CPLoop/3, CP_count_scope/3
  ChannelOut/3 -> dout/1
  ChannelOut/2 -> cout/1
  ChannelOut/1 -> vout/1
  ChannelIn/2 -> CP_count_scope/8
  And1/1 -> ChannelOut/1
  CPLen/1 -> ChannelIn/4
  FFTSize/1 -> ChannelIn/5
  ChannelIn/5 -> ChannelOut/4, LShift1/2
  NumberOfFFTs/1 -> ChannelIn/6
  chin/1 -> ChannelIn/2
  din/1 -> ChannelIn/3
  vin/1 -> ChannelIn/1
  ChannelIn/6 -> Convert/1
  ChannelIn/4 -> CP_count_scope/2, Mux1/1, Display1/1
  ChannelIn/7 -> CP_count_scope/1, CPLoop/1
  SOP/1 -> ChannelIn/7
  FFTLoop/1 -> And1/1, FFT_sample_count_scope/4
  Mux/1 -> FFT_sample_count_scope/2, FFTLoop/2
  CPLoop/4 -> CP_count_scope/7, Demux/1, FFT_sample_count_scope/1
  FFTLoop/2 -> Demux1/1, FFT_sample_count_scope/5
  FFTLoop/3 -> FFT_sample_count_scope/6
  FFTLoop/4 -> FFT_sample_count_scope/7
  CPLoop/1 -> CP_count_scope/4
  CPLoop/2 -> CP_count_scope/5
  CPLoop/3 -> CP_count_scope/6
  Const3/1 -> LShift1/1
  LShift1/1 -> Mux/2, Display3/1
  Convert/1 -> Mux/1
  Const1/1 -> Mux/3
  Mux1/1 -> CPLoop/2
  Const2/1 -> Mux1/2
  And/1 -> SampleDelay/1
  Demux/2 -> And/2
  Demux/1 -> And/1
  ChannelOut/5 -> qSOP/1
  ChannelOut/4 -> qFFTSize/1
  BW/10/1 -> ChannelIn/8
  ChannelOut/6 -> qBWby10/1
  ChannelIn/8 -> ChannelOut/6
  SampleDelay/1 -> ChannelOut/5, FFTLoop/1
  Demux1/3 -> Convert1/1, FFT_sample_count_scope/8
  Demux1/1 -> Terminator1/1
  Demux1/2 -> Terminator/1
  Convert1/1 -> ChannelOut/2
  ChannelIn/3 -> ChannelOut/3, FFT_sample_count_scope/9
  TimeReference/1 -> ChannelIn/9
  ChannelIn/9 -> ChannelOut/7
  ChannelOut/7 -> T_ref/1

== system prach_shortFormat_fftShift/prach/PRACH_CC/ScaleAndSelect ==
  vin : Inport
  chin : Inport  Port=2
  FFTSize : Inport  Port=3
  d : Inport  Port=4
  BWby10 : Inport  Port=5
  TimeReference : Inport  Port=6
  And : DSPBAPrim/And  primtype=and  nInputs=2  nOutputs=1  omode=Inherit via internal rule  otype=sfix(16)  scale=2^-15  rndmethod=Unbiased  factor=1  satmethod=Symmetric  shift_vec=[0 1 2 -1]  value=0  inPortNames=[' '; ' '; ' '; ' '; ' '; ' '; ' '; ' '; ' '; ' '; ' '; ' '; ' '; ' '; ' '; ' '; ]  outPortNames=[' ']  dspbaimage=dspba_prim.svg  text=fprintf('&');  style=Optimised  visibilities=8+2  version=20211007
  And1 : DSPBAPrim/And  primtype=and  nInputs=2  nOutputs=1  omode=Inherit via internal rule  otype=sfix(16)  scale=2^-15  rndmethod=Unbiased  factor=1  satmethod=Symmetric  shift_vec=[0 1 2 -1]  value=0  inPortNames=[' '; ' '; ' '; ' '; ' '; ' '; ' '; ' '; ' '; ' '; ' '; ' '; ' '; ' '; ' '; ' '; ]  outPortNames=[' ']  dspbaimage=dspba_prim.svg  text=fprintf('&');  style=Optimised  visibilities=8+2  version=20211007
  ChannelIn : DSPBAPrim/ChannelIn  primtype=channelin  nInputs=dspba_internal_get_channel_ports(gcb)  nOutputs=dspba_internal_get_channel_ports(gcb)  omode=Inherit via internal rule  otype=sfix(16)  scale=2^-15  rndmethod=Unbiased  factor=1  satmethod=Symmetric  shift_vec=[0 1 2 -1]  value=4  inPortNames=['v'; 'c'; '0'; '1'; '2'; '3'; '4'; '5'; '6'; '7'; '8'; '9'; 'A'; 'B'; 'D'; 'E'; 'F'; 'G'; 'H'; 'I'; 'J'; 'K'; 'L'; 'M'; 'N'; 'O'; 'P'; 'Q'; 'R'; 'S'; 'T'; 'U'; 'W'; 'X'; 'Y'; 'Z']  outPortNames=['v'; 'c'; '0'; '1'; '2'; '3'; '4'; '5'; '6'; '7'; '8'; '9'; 'A'; 'B'; 'D'; 'E'; 'F'; 'G'; 'H'; 'I'; 'J'; 'K'; 'L'; 'M'; 'N'; 'O'; 'P'; 'Q'; 'R'; 'S'; 'T'; 'U'; 'W'; 'X'; 'Y'; 'Z']  dspbaimage=dspba_prim_channel_tall.svg  text=fprintf('In');  style=Optimised  dataSignals=4  foldingEnabled=off  channels=1  sampleRate=200  packetBeginPresent=off  packetBeginEnabled=off  visibilities=dspba_ChannelInVis(gcb)  scheduleOrigin=on  version=20211214
  ChannelOut : DSPBAPrim/ChannelOut  primtype=channelout  nInputs=dspba_internal_get_channel_ports(gcb)  nOutputs=dspba_internal_get_channel_ports(gcb)  omode=Inherit via internal rule  otype=sfix(16)  scale=2^-15  rndmethod=Unbiased  factor=1  satmethod=Symmetric  shift_vec=[0 1 2 -1]  value=3  inPortNames=['v'; 'c'; '0'; '1'; '2'; '3'; '4'; '5'; '6'; '7'; '8'; '9'; 'A'; 'B'; 'D'; 'E'; 'F'; 'G'; 'H'; 'I'; 'J'; 'K'; 'L'; 'M'; 'N'; 'O'; 'P'; 'Q'; 'R'; 'S'; 'T'; 'U'; 'W'; 'X'; 'Y'; 'Z']  outPortNames=['v'; 'c'; '0'; '1'; '2'; '3'; '4'; '5'; '6'; '7'; '8'; '9'; 'A'; 'B'; 'D'; 'E'; 'F'; 'G'; 'H'; 'I'; 'J'; 'K'; 'L'; 'M'; 'N'; 'O'; 'P'; 'Q'; 'R'; 'S'; 'T'; 'U'; 'W'; 'X'; 'Y'; 'Z']  dspbaimage=dspba_prim_channel_tall.svg  text=fprintf('Out%s', AdvDSPBChannelOutDisplay(latency));  style=Optimised  dataSignals=3  foldingEnabled=off  channels=1  sampleRate=200  packetBeginPresent=off  packetBeginEnabled=off  visibilities=dspba_ChannelOutVis(gcb)  latency=6  version=20211214
  ChannelOut1 : DSPBAPrim/ChannelOut  primtype=channelout  nInputs=dspba_internal_get_channel_ports(gcb)  nOutputs=dspba_internal_get_channel_ports(gcb)  omode=Inherit via internal rule  otype=sfix(16)  scale=2^-15  rndmethod=Unbiased  factor=1  satmethod=Symmetric  shift_vec=[0 1 2 -1]  value=2  inPortNames=['v'; 'c'; '0'; '1'; '2'; '3'; '4'; '5'; '6'; '7'; '8'; '9'; 'A'; 'B'; 'D'; 'E'; 'F'; 'G'; 'H'; 'I'; 'J'; 'K'; 'L'; 'M'; 'N'; 'O'; 'P'; 'Q'; 'R'; 'S'; 'T'; 'U'; 'W'; 'X'; 'Y'; 'Z']  outPortNames=['v'; 'c'; '0'; '1'; '2'; '3'; '4'; '5'; '6'; '7'; '8'; '9'; 'A'; 'B'; 'D'; 'E'; 'F'; 'G'; 'H'; 'I'; 'J'; 'K'; 'L'; 'M'; 'N'; 'O'; 'P'; 'Q'; 'R'; 'S'; 'T'; 'U'; 'W'; 'X'; 'Y'; 'Z']  dspbaimage=dspba_prim_channel_tall.svg  text=fprintf('Out%s', AdvDSPBChannelOutDisplay(latency));  style=Optimised  dataSignals=2  foldingEnabled=off  channels=1  sampleRate=200  packetBeginPresent=off  packetBeginEnabled=off  visibilities=dspba_ChannelOutVis(gcb)  latency=12  version=20211214
  CmpEQ : DSPBAPrim/CmpEQ  primtype=cmpeq  nInputs=2  nOutputs=1  omode=boolean  otype=sfix(16)  scale=2^-15  rndmethod=Unbiased  factor=1  satmethod=Symmetric  shift_vec=[0 1 2 -1]  value=0  inPortNames=[' '; ' ';]  outPortNames=[' ']  dspbaimage=dspba_prim.svg  text=fprintf('==');  style=Optimised  visibilities=0  advOptions=[]  version=20211007
  Const : DSPBAPrim/Const  primtype=const  nInputs=0  nOutputs=1  omode=Specify via dialog  otype=uint(8);  scale=2^0  rndmethod=Unbiased  factor=1  satmethod=Symmetric  shift_vec=[0 1 2 -1]  value=0  inPortNames=['+'; '+';]  outPortNames=[' ']  dspbaimage=dspba_prim.svg  text=fprintf('%s', num2str(value));  style=Optimised  visibilities=8 + 1024  floatPrecision=float32_m23  warnSaturation=on  version=20211007  SampleTime=inf
  FFT Shift : Subsystem
  IndexCounter : Subsystem
  ScaleOutputAndCheck : Subsystem
      mask Display:
      | color('w');image('dspba_prim.jpg');
      | fprintf('*2^PRACH_fft_scale');
      | port_label('input',1,'din');
      | port_label('output',1,'dout');
  Sub : DSPBAPrim/Sub  primtype=sub  nInputs=2  nOutputs=1  omode=Inherit via internal rule with word growth  otype=sfix(16)  scale=2^-15  rndmethod=Unbiased  factor=1  satmethod=Symmetric  shift_vec=[0 1 2 -1]  value=0  inPortNames=['+'; '-';]  outPortNames=[' ']  dspbaimage=dspba_prim.svg  text=fprintf('-');  style=Optimised  visibilities=8+2^17+2^18  floatRounding=correct  advOptions=[]  version=20211007
  SynthesisInfo : DSPBAPrim/SynthesisInfo  primtype=synthinfo  nInputs=0  nOutputs=0  omode=Inherit via internal rule  otype=sfix(16)  scale=2^-15  rndmethod=Truncate  factor=1  satmethod=Symmetric  shift_vec=[0 1 2 -1]  value=99  inPortNames=[' '; ' ';]  outPortNames=[' ']  dspbaimage=dspba_prim_ctrl.jpg  text=fprintf('Style=%s', style);  style=Scheduled  visibilities=2^17+2^18+2^19+2^20+2^21+2^22+2^23+2^24  constraintPair=None  constraintRelation=>  constraintLimit=6  modelRefSign=+  modelRef=''  showSchedule=off  simulationMode=Use Global Value  resetMinimization=Conditional - On for ChannelIn/Out only  version=20220106
  gen_139_valids : Subsystem
  latch_0L : DSPBAControl/latch_0L
  qv : Outport  VectorParamsAs1DForOutWhenUnconnected=off
  qch : Outport  Port=2  VectorParamsAs1DForOutWhenUnconnected=off
  q : Outport  Port=3  VectorParamsAs1DForOutWhenUnconnected=off
  qv139 : Outport  Port=4  VectorParamsAs1DForOutWhenUnconnected=off
  FreqBinIdx : Outport  Port=5  VectorParamsAs1DForOutWhenUnconnected=off
  vout_FFTshift : Outport  Port=6  VectorParamsAs1DForOutWhenUnconnected=off
  cout_FFTshift : Outport  Port=7  VectorParamsAs1DForOutWhenUnconnected=off
  dout_FFTshift : Outport  Port=8  VectorParamsAs1DForOutWhenUnconnected=off
  Tref : Outport  Port=9  VectorParamsAs1DForOutWhenUnconnected=off
  wires:
  gen_139_valids/2(startSymFD) -> Sub/2
  ChannelIn/3 -> IndexCounter/2(FFTSize), gen_139_valids/2(FFTSize)
  ChannelIn/5 -> gen_139_valids/3(BWby10)
  gen_139_valids/1(v139) -> And1/2
  IndexCounter/1(index) -> gen_139_valids/1(Index), Sub/1
  BWby10/1 -> ChannelIn/5
  ChannelOut/5 -> FreqBinIdx/1
  ChannelIn/4 -> ScaleOutputAndCheck/1(din)
  d/1 -> ChannelIn/4
  FFTSize/1 -> ChannelIn/3
  ChannelOut/4 -> qv139/1
  ChannelOut/3 -> q/1
  chin/1 -> ChannelIn/2
  vin/1 -> ChannelIn/1
  ChannelIn/1 -> IndexCounter/1(v), And1/1, ChannelOut/1, And/2
  ChannelOut/2 -> qch/1
  ChannelOut/1 -> qv/1
  ChannelIn/2 -> CmpEQ/2, ChannelOut/2, FFT Shift/1(ch_in)
  ChannelOut1/2 -> cout_FFTshift/1
  ChannelOut1/3 -> dout_FFTshift/1
  And1/1 -> FFT Shift/3(v_in), ChannelOut/4
  ChannelOut1/1 -> vout_FFTshift/1
  ScaleOutputAndCheck/1(dout) -> FFT Shift/2(din), ChannelOut/3
  Sub/1 -> FFT Shift/4(WR_add), ChannelOut/5
  FFT Shift/1(v) -> ChannelOut1/1
  FFT Shift/2(q) -> ChannelOut1/3
  TimeReference/1 -> ChannelIn/6
  ChannelIn/6 -> latch_0L/2
  ChannelOut1/4 -> Tref/1
  Const/1 -> CmpEQ/1
  CmpEQ/1 -> And/1
  And/1 -> latch_0L/1
  latch_0L/1 -> ChannelOut1/4
  FFT Shift/3(c) -> ChannelOut1/2

== system prach_shortFormat_fftShift/prach/PRACH_CC/Stream2BlockConv ==
  vin : Inport
  chin : Inport  Port=2
  din : Inport  Port=3
  FFTSize : Inport  Port=4
  SOP : Inport  Port=5
  BWby10 : Inport  Port=6
  TimeReference : Inport  Port=7
  ChannelIn : DSPBAPrim/ChannelIn  primtype=channelin  nInputs=dspba_internal_get_channel_ports(gcb)  nOutputs=dspba_internal_get_channel_ports(gcb)  omode=Inherit via internal rule  otype=sfix(16)  scale=2^-15  rndmethod=Unbiased  factor=1  satmethod=Symmetric  shift_vec=[0 1 2 -1]  value=5  inPortNames=['v'; 'c'; '0'; '1'; '2'; '3'; '4'; '5'; '6'; '7'; '8'; '9'; 'A'; 'B'; 'D'; 'E'; 'F'; 'G'; 'H'; 'I'; 'J'; 'K'; 'L'; 'M'; 'N'; 'O'; 'P'; 'Q'; 'R'; 'S'; 'T'; 'U'; 'W'; 'X'; 'Y'; 'Z']  outPortNames=['v'; 'c'; '0'; '1'; '2'; '3'; '4'; '5'; '6'; '7'; '8'; '9'; 'A'; 'B'; 'D'; 'E'; 'F'; 'G'; 'H'; 'I'; 'J'; 'K'; 'L'; 'M'; 'N'; 'O'; 'P'; 'Q'; 'R'; 'S'; 'T'; 'U'; 'W'; 'X'; 'Y'; 'Z']  dspbaimage=dspba_prim_channel_tall.svg  text=fprintf('In');  style=Optimised  dataSignals=5  foldingEnabled=off  channels=1  sampleRate=200  packetBeginPresent=off  packetBeginEnabled=off  visibilities=dspba_ChannelInVis(gcb)  scheduleOrigin=on  version=20211214
  ChannelOut : DSPBAPrim/ChannelOut  primtype=channelout  nInputs=dspba_internal_get_channel_ports(gcb)  nOutputs=dspba_internal_get_channel_ports(gcb)  omode=Inherit via internal rule  otype=sfix(16)  scale=2^-15  rndmethod=Unbiased  factor=1  satmethod=Symmetric  shift_vec=[0 1 2 -1]  value=4  inPortNames=['v'; 'c'; '0'; '1'; '2'; '3'; '4'; '5'; '6'; '7'; '8'; '9'; 'A'; 'B'; 'D'; 'E'; 'F'; 'G'; 'H'; 'I'; 'J'; 'K'; 'L'; 'M'; 'N'; 'O'; 'P'; 'Q'; 'R'; 'S'; 'T'; 'U'; 'W'; 'X'; 'Y'; 'Z']  outPortNames=['v'; 'c'; '0'; '1'; '2'; '3'; '4'; '5'; '6'; '7'; '8'; '9'; 'A'; 'B'; 'D'; 'E'; 'F'; 'G'; 'H'; 'I'; 'J'; 'K'; 'L'; 'M'; 'N'; 'O'; 'P'; 'Q'; 'R'; 'S'; 'T'; 'U'; 'W'; 'X'; 'Y'; 'Z']  dspbaimage=dspba_prim_channel_tall.svg  text=fprintf('Out%s', AdvDSPBChannelOutDisplay(latency));  style=Optimised  dataSignals=4  foldingEnabled=off  channels=1  sampleRate=200  packetBeginPresent=off  packetBeginEnabled=off  visibilities=dspba_ChannelOutVis(gcb)  latency=6  version=20211214
  Convert3 : DSPBAPrim/Convert  primtype=convert  nInputs=1  nOutputs=1  omode=Specify via dialog  otype=uint(8)  scale=1  rndmethod=Truncate  factor=1  satmethod=None  shift_vec=[0 1 2 -1]  value=round([0:255]/17)  inPortNames=[' '; ' ';]  outPortNames=[' '; 'c']  dspbaimage=dspba_prim_wide.svg  text=fprintf('convert');  style=Optimised  visibilities=8+64+256+2^17  clipdetect=off  floatPrecision=float32_m23  advOptions=[]  version=20211007
  MemArray : DSPBAPrim/DualMem  primtype=dualmem  nInputs=4  nOutputs=2  omode=Inherit via internal rule  otype=sfix(16)  scale=2^-15  rndmethod=Unbiased  factor=1  satmethod=Symmetric  shift_vec=[0 1 2 -1]  value=[zeros(NFftMax*2, NAnts)]  inPortNames=['d1'; 'a1'; 'w1'; 'a2']  outPortNames=['q1'; 'q2']  dspbaimage=dspba_prim_tall.svg  text=fprintf('dmem%s',AdvDSPBDMemDisplay(UseDontCare));  style=Optimised  visibilities=8 + 1024 + 2^17 + 2^18  UseDontCare=on  TwinWritePorts=off  init=on  ProvideReadAccess=off  version=20211007
  RdAddrGen : Subsystem  mask{NAnts=NAnts, NFftMax=NFftMax}
      mask prompts: NAnts "Number of Antennas"; NFftMax "Maximum FFT size"
  SampleDelay : DSPBAPrim/SampleDelay  primtype=sampdelay  nInputs=1  nOutputs=1  omode=Inherit via internal rule  otype=sfix(16)  scale=2^-15  rndmethod=Unbiased  factor=1  satmethod=Symmetric  shift_vec=[0 1 2 -1]  floatPrecision=float32_m23  value=1  inPortNames=[' '; ' ';]  outPortNames=[' ']  dspbaimage=dspba_prim.svg  text=dpoly(1, eye(1,value+1), 'z')  style=Optimised  visibilities=8 + 1024 + 2^17 + 2^18  flexible=off  slackgroup=0  augmented=0  version=20211007  advOptions=[]
  Stream2BlockScope : Scope  NumInputPorts=6
  SynthesisInfo : DSPBAPrim/SynthesisInfo  primtype=synthinfo  nInputs=0  nOutputs=0  omode=Inherit via internal rule  otype=sfix(16)  scale=2^-15  rndmethod=Truncate  factor=1  satmethod=Symmetric  shift_vec=[0 1 2 -1]  value=99  inPortNames=[' '; ' ';]  outPortNames=[' ']  dspbaimage=dspba_prim_ctrl.jpg  text=fprintf('Style=%s', style);  style=Scheduled  visibilities=2^17+2^18+2^19+2^20+2^21+2^22+2^23+2^24  constraintPair=None  constraintRelation=>  constraintLimit=6  modelRefSign=+  modelRef=''  showSchedule=off  simulationMode=Use Global Value  resetMinimization=Conditional - On for ChannelIn/Out only  version=20220106
  Terminator1 : Terminator
  Terminator4 : Terminator
  Vector Mux : DSPBAVectorUtil/Vector Mux  vecWidth=NAnts
  WrCtrl : Subsystem  mask{NAnts=NAnts, NFftMax=NFftMax}
      mask prompts: NAnts "Number of Antennas"; NFftMax "Maximum FFT size"
  latch_0L : DSPBAControl/latch_0L
  latch_0L1 : DSPBAControl/latch_0L
  vout : Outport  VectorParamsAs1DForOutWhenUnconnected=off
  cout : Outport  Port=2  VectorParamsAs1DForOutWhenUnconnected=off
  qFFTSize : Outport  Port=3  VectorParamsAs1DForOutWhenUnconnected=off
  q : Outport  Port=4  VectorParamsAs1DForOutWhenUnconnected=off
  qBWby10 : Outport  Port=5  VectorParamsAs1DForOutWhenUnconnected=off
  Tref : Outport  Port=6  VectorParamsAs1DForOutWhenUnconnected=off
  wires:
  ChannelOut/1 -> vout/1
  ChannelOut/2 -> cout/1
  vin/1 -> ChannelIn/1
  chin/1 -> ChannelIn/2
  din/1 -> ChannelIn/3
  ChannelIn/1 -> WrCtrl/1(vin)
  RdAddrGen/2(AntAddr) -> Vector Mux/2, Convert3/1, Stream2BlockScope/5  "antenna_rd_addr"
  ChannelIn/3 -> Stream2BlockScope/1, MemArray/1  "data_in"
  MemArray/2 -> Vector Mux/1
  Vector Mux/1 -> Stream2BlockScope/6, ChannelOut/4  "data_out"
  MemArray/1 -> Terminator4/1
  latch_0L/1 -> WrCtrl/2(FFTSize), latch_0L1/2
  latch_0L1/1 -> ChannelOut/3, RdAddrGen/2(FFTSize)
  RdAddrGen/1(FFtPntAddr) -> MemArray/4, Stream2BlockScope/4  "sample_rd_addr"
  Convert3/1 -> ChannelOut/2
  WrCtrl/1(WrAddr) -> MemArray/2, Stream2BlockScope/2  "wr_addr"
  WrCtrl/2(wr) -> MemArray/3, Stream2BlockScope/3  "wr"
  WrCtrl/3(FirstBlkRdy) -> latch_0L1/1, SampleDelay/1
  RdAddrGen/3(Rd) -> ChannelOut/1
  ChannelIn/2 -> Terminator1/1
  FFTSize/1 -> ChannelIn/4
  SOP/1 -> ChannelIn/5
  ChannelIn/4 -> latch_0L/2
  ChannelIn/5 -> latch_0L/1, WrCtrl/3(go)
  ChannelOut/3 -> qFFTSize/1
  ChannelOut/4 -> q/1
  BWby10/1 -> ChannelIn/6
  ChannelOut/5 -> qBWby10/1
  ChannelIn/6 -> ChannelOut/5
  SampleDelay/1 -> RdAddrGen/1(go)
  WrCtrl/4(BankRdy) -> RdAddrGen/3(gobank)
  TimeReference/1 -> ChannelIn/7
  ChannelIn/7 -> ChannelOut/6
  ChannelOut/6 -> Tref/1
